simulink model "WaterProp"  (R2013b)
settings: Solver=FixedStepDiscrete  StartTime=0.0  StopTime=19.5  FixedStep=1  MaxStep=1  RelTol=1e-3
libraries: simulink x2
settings Model: Creator=awohlfei  LastModifiedBy=drhf
settings DataIOCC: SignalLoggingSaveFormat=ModelDataLogs  SaveTime=off
settings OptimizationCC: ExpressionDepthLimit=2147483647
settings DebuggingCC: FcnCallInpInsideContextMsg=EnableAllAsWarning  FrameProcessingCompatibilityMsg=error  StateNameClashWarn=warning
settings GRTTargetCC: CodeReplacementLibrary=C89/C90 (ANSI)

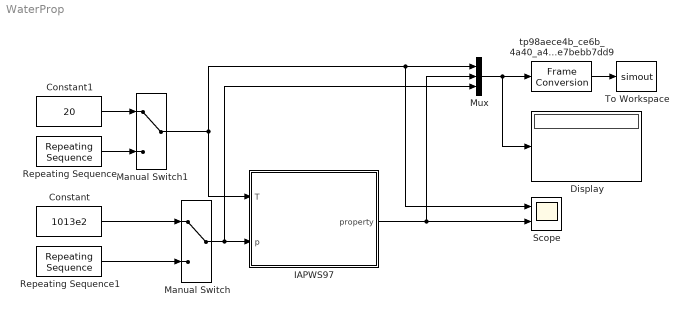
== system WaterProp ==
  Constant : Constant  Value=1013e2
  Constant1 : Constant  Value=20
  Display : Display
  IAPWS97 : Subsystem  mask{PROPERTY=TEMPERATURE_CONDUCTIVITY}
      mask TypeOptions PROPERTY: DENSITY | HEAT_CAPACITY | THERMAL_CONDUCTIVITY | VISCOSITY | ENTHALPY | ENTROPY | PRANDTL | SPECIFIC_VOLUME | EVAPORATION_ENTHALPY | VAPOURPRESSURE | SATURATIONTEMPERATURE | SATURATIONPROPERTY | TEMPERATURE_CONDUCTIVITY | ENTHALPY2TEMPERATURE
  Manual Switch : ManualSwitch
  Manual Switch1 : ManualSwitch
  Mux : Mux  Inputs=3
  Repeating Sequence : simulink/Sources/Repeating Sequence  rep_seq_t=[0 19 21]  rep_seq_y=[10 200 200]
  Repeating Sequence1 : simulink/Sources/Repeating Sequence  rep_seq_t=[0 19 21]  rep_seq_y=[1 3e5 3e5]
  Scope : Scope  NumInputPorts=2
      settings: YMin=-25.00000~-5  YMax=225.00000~5
  To Workspace : ToWorkspace  VariableName=simout  SampleTime=1
  tp98aece4b_ce6b_4a40_a4f5_b9e7bebb7dd9 : FrameConversion  OutFrame=Sample-based
  wires:
  Manual Switch1/1 -> IAPWS97/1(T), Scope/1, Mux/1
  IAPWS97/1(property) -> Mux/2, Scope/2
  Constant/1 -> Manual Switch/1
  Repeating Sequence1/1 -> Manual Switch/2
  Manual Switch/1 -> Mux/3, IAPWS97/2(p)
  Mux/1 -> Display/1, tp98aece4b_ce6b_4a40_a4f5_b9e7bebb7dd9/1
  tp98aece4b_ce6b_4a40_a4f5_b9e7bebb7dd9/1 -> To Workspace/1
  Repeating Sequence/1 -> Manual Switch1/2
  Constant1/1 -> Manual Switch1/1

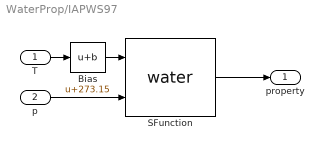
== system WaterProp/IAPWS97 ==
  T : Inport
  p : Inport  Port=2
  Bias : Bias  Bias=273.15
  SFunction : S-Function  FunctionName=water  Parameters=PROPERTY  EnableBusSupport=off
  property : Outport
  wires:
  T/1 -> Bias/1
  p/1 -> SFunction/2
  SFunction/1 -> property/1
  Bias/1 -> SFunction/1
